simulink model "w2problem3"  (R2020b)
settings: Solver=ode45  StartTime=0.0  StopTime=120  RelTol=1e-3
model workspace (MAT data in the model file):
  Kd = Simulink.Parameter
  Kd.Value = 1
  Kd.DataType = 'auto'
  Kd.Dimensions = [1 1]
  Ki = Simulink.Parameter
  Ki.Value = 1
  Ki.DataType = 'auto'
  Ki.Dimensions = [1 1]
  Kp = Simulink.Parameter
  Kp.Value = 1
  Kp.DataType = 'auto'
  Kp.Dimensions = [1 1]
  b = Simulink.Parameter
  b.Value = 50
  b.DataType = 'auto'
  b.Dimensions = [1 1]
  m = Simulink.Parameter
  m.Value = 1000
  m.DataType = 'auto'
  m.Dimensions = [1 1]
  u = Simulink.Parameter
  u.Value = 500
  u.DataType = 'auto'
  u.Dimensions = [1 1]
settings Model: DataDictionary=w2pr3_data.sldd  Creator=k.Raviteja  LastModifiedBy=k.Raviteja

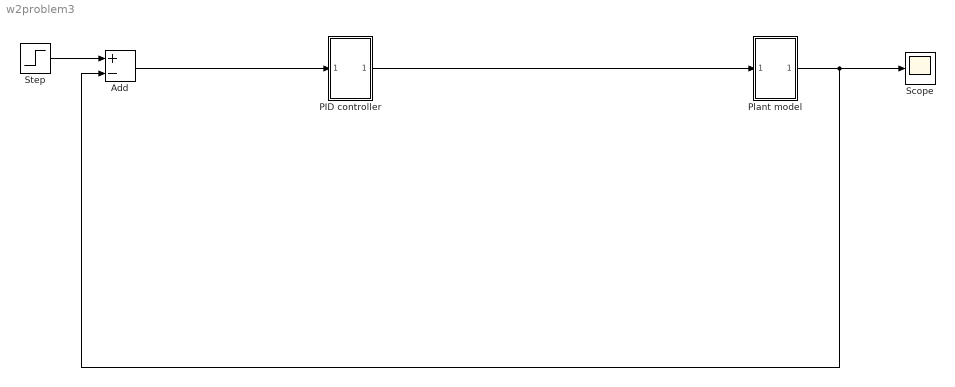
== system w2problem3 ==
  Add : Sum  Inputs=+-
  PID controller : ModelReference  ModelNameDialog=PID_controller  SimulationMode=Normal  ModelReferenceVersion=1.4
  Plant model : Subsystem
  Scope : Scope
  Step : Step  Time=0  After=u  SampleTime=0
  wires:
  Plant model/1(Out1) -> Add/2, Scope/1
  Step/1 -> Add/1
  Add/1 -> PID controller/1
  PID controller/1 -> Plant model/1(In1)

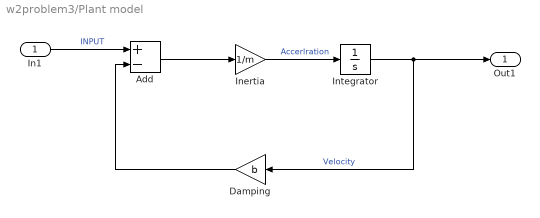
== system w2problem3/Plant model ==
  In1 : Inport
  Add : Sum  Inputs=+-
  Damping : Gain  Gain=b
  "Inertia " : Gain  Gain=1/m
  Integrator : Integrator
  Out1 : Outport
  wires:
  In1/1 -> Add/1  "INPUT"
  Integrator/1 -> Out1/1, Damping/1  "Velocity"
  Add/1 -> "Inertia "/1
  Damping/1 -> Add/2
  "Inertia "/1 -> Integrator/1  "Accerlration"
